simulink library "lib_GenTools_WeightedAveraging"  (R2015a)
settings: Solver=ode45  StartTime=0.0  StopTime=10.0  RelTol=1e-3
settings Model: Creator=jlkratz  LastModifiedBy=jlkratz

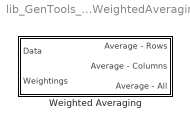
== system lib_GenTools_WeightedAveraging ==
  Weighted Averaging : Subsystem  mask(TSAT: Weighted Averaging Block){avg_rows_M=on, avg_cols_M=on, avg_all_M=on, BN_M=gcb}
      mask prompts: avg_rows_M "avg_rows_M - Average Rows"; avg_cols_M "avg_cols_M - Average Columns"; avg_all_M "avg_all_M - Average All"; BN_M "BN_M - Block Name"
      mask help: This block is meant for weighted averaging 1-D and 2-D arrays. It can be used to return the average of the rows, columns, or all values within the data set.
      mask init:
      | % Setup Outports ---------------------------------------------------------%
      | 
      | % Outport Numbers
      | n = 1; %first inport
      | 
      | % Average Rows Inport
      | if avg_rows_M == 1
      |     if strcmp(get_param([BN_M '/Average - Rows'],'BlockType'),'Terminator')
      |         MSK_ReplaceBlock_TSAT([BN_M '/Average - Rows'],'built-in/Outport');
      |     end
      |     set_param([BN_M '/Average - Rows'],'Port',num2str(n));
      |     n = n + 1;
      | elseif avg_rows_M == 0
      |     if strcmp(get_param([BN_M '/Average - Rows'],'BlockType'),'Outport')
      |         MSK_ReplaceBlock_TSAT([BN_M '/Average - Rows'],'built-in/Terminator');
      |     end
      | end
      | 
      | % Average Columns Inport
      | if avg_cols_M == 1
      |     if strcmp(get_param([BN_M '/Average - Columns'],'BlockType'),'Terminator')
      |         MSK_ReplaceBlock_TSAT([BN_M '/Average - Columns'],'built-in/Outport');
      |     end
      |     set_param([BN_M '/Average - Columns'],'Port',num2str(n));
      |     n = n + 1;
      | elseif avg_cols_M == 0
      |     if strcmp(get_param([BN_M '/Average - Columns'],'BlockType'),'Outport')
      |         MSK_ReplaceBlock_TSAT([BN_M '/Average - Columns'],'built-in/Terminator');
      |     end
      | end
      | 
      | % Average All Inport
      | if avg_all_M == 1
      |     if strcmp(get_param([BN_M '/Average - All'],'BlockType'),'Terminator')
      |         MSK_ReplaceBlock_TSAT([BN_M '/Average - All'],'built-in/Outport');
      |     end
      |     set_param([BN_M '/Average - All'],'Port',num2str(n));
      |     n = n + 1;
      | elseif avg_all_M == 0
      |     if strcmp(get_param([BN_M '/Average - All'],'BlockType'),'Outport')
      |         MSK_ReplaceBlock_TSAT([BN_M '/Average - All'],'built-in/Terminator');
      |     end
      | end
      mask Help: web(which('GenTools_TSAT_WeightedAveraging.html'),'-helpbrowser')

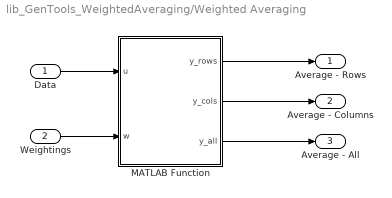
== system lib_GenTools_WeightedAveraging/Weighted Averaging ==
  Data : Inport
  Weightings : Inport  Port=2
  MATLAB Function : MATLAB Function  TreatAsAtomicUnit=on
  Average - Rows : Outport
  Average - Columns : Outport  Port=2
  Average - All : Outport  Port=3
  wires:
  MATLAB Function/3(y_all) -> Average - All/1
  MATLAB Function/2(y_cols) -> Average - Columns/1
  MATLAB Function/1(y_rows) -> Average - Rows/1
  Data/1 -> MATLAB Function/1(u)
  Weightings/1 -> MATLAB Function/2(w)

== matlab function lib_GenTools_WeightedAveraging/Weighted Averaging/MATLAB Function ==
  data: u input; y_rows output; y_cols output; y_all output; w input
function [y_rows, y_cols, y_all] = average(u,w)
%#codegen

[n,m] = size(u);

%average rows
y_rows = zeros(n,1);
for i = 1:n
    y_rows(i) = sum(u(i,:).*w(i,:))/sum(w(i,:));
end

%average columns
y_cols = zeros(1,m);
for j = 1:m
    y_cols(j) = sum(u(:,j).*w(:,j))/sum(w(:,j));
end
    
%average all   
SUM1 = 0;
SUM2 = 0;
for i = 1:n
    for j = 1:m
        SUM1 = SUM1 + u(i,j).*w(i,j);
        SUM2 = SUM2 + w(i,j);
    end
end
y_all = SUM1/SUM2;
